simulink library "tetherBuoyAndWeight_ul"  (R2018b)
settings: Solver=VariableStepAuto  StartTime=0.0  StopTime=10.0  RelTol=1e-3
values from neighbouring files (symbols this model uses):
  rho_fluid = 1000    [tetherBuoyAndWeight_ts.m]
  rho_tether = 1010    [tetherBuoyAndWeight_ts.m]
libraries: cylinderVolume_ul x1
settings Model: Creator=asiddiq2  LastModifiedBy=asiddiq2

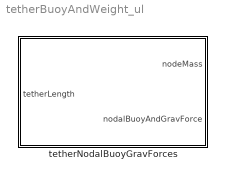
== system tetherBuoyAndWeight_ul ==
  tetherNodalBuoyGravForces : Subsystem  mask{rhoFluid=rho_fluid, gravAccl=10, numNode=4, diaTether=1, rhoTether=rho_tether}
      mask prompts: rhoFluid "Fluid density"; gravAccl "Gravitational acceleration"; numNode "Number of nodes"; diaTether "Tether diameter"; rhoTether "Tether density"
      mask DialogControl Container3 Prompt: Environment
      mask DialogControl ParameterGroupVar Prompt: Tether

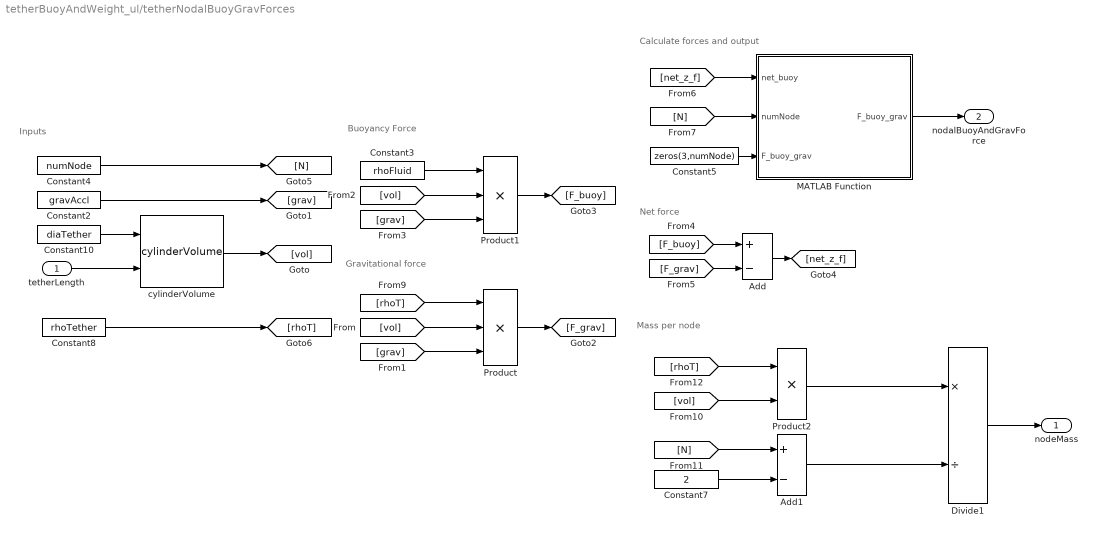
== system tetherBuoyAndWeight_ul/tetherNodalBuoyGravForces ==
  note: Inputs
  note: Calculate forces and output
  note: Mass per node
  note: Net force
  note: Buoyancy Force
  note: Gravitational force
  tetherLength : Inport  PortDimensions=[1,1]
  Add : Sum  Inputs=+-
  Add1 : Sum  Inputs=+-
  Constant10 : Constant  Value=diaTether  VectorParams1D=off
  Constant2 : Constant  Value=gravAccl  VectorParams1D=off
  Constant3 : Constant  Value=rhoFluid  VectorParams1D=off
  Constant4 : Constant  Value=numNode  VectorParams1D=off
  Constant5 : Constant  Value=zeros(3,numNode)  VectorParams1D=off
  Constant7 : Constant  Value=2
  Constant8 : Constant  Value=rhoTether  VectorParams1D=off
  Divide1 : Product  Inputs=*/
  MATLAB Function : MATLAB Function  TreatAsAtomicUnit=on
  Product : Product  Inputs=3
  Product1 : Product  Inputs=3
  Product2 : Product
  cylinderVolume : cylinderVolume_ul/cylinderVolume  SystemSampleTime=-1
  nodeMass : Outport
  nodalBuoyAndGravForce : Outport  Port=2
  wires:
  tetherLength/1 -> cylinderVolume/2
  cylinderVolume/1 -> [vol]
  Constant2/1 -> [grav]
  [rhoT] -> Product/1
  [vol] -> Product/2
  [grav] -> Product/3
  Product/1 -> [F_grav]
  [grav] -> Product1/3
  Constant3/1 -> Product1/1
  [vol] -> Product1/2
  Product1/1 -> [F_buoy]
  [F_buoy] -> Add/1
  [F_grav] -> Add/2
  Add/1 -> [net_z_f]
  [net_z_f] -> MATLAB Function/1(net_buoy)
  Constant4/1 -> [N]
  [N] -> MATLAB Function/2(numNode)
  Constant5/1 -> MATLAB Function/3("F_buoy_grav ")
  [vol] -> Product2/2
  [rhoT] -> Product2/1
  Product2/1 -> Divide1/1
  Divide1/1 -> nodeMass/1
  [N] -> Add1/1
  Add1/1 -> Divide1/2
  Constant7/1 -> Add1/2
  Constant10/1 -> cylinderVolume/1
  Constant8/1 -> [rhoT]
  MATLAB Function/1(F_buoy_grav) -> nodalBuoyAndGravForce/1

== matlab function tetherBuoyAndWeight_ul/tetherNodalBuoyGravForces/MATLAB Function ==
  data: net_buoy input; F_buoy_grav output; numNode input; F_buoy_grav input
function F_buoy_grav = fcn(net_buoy,numNode,F_buoy_grav)

for ii = 1:numNode
    if ii == 1
        F_buoy_grav(:,ii) = zeros(3,1);
    elseif ii>1 && ii<numNode
        F_buoy_grav(:,ii) = net_buoy/(numNode-2)*[0; 0; 1];
    elseif ii == numNode
        F_buoy_grav(:,ii) = zeros(3,1);
    end
    
end

end
